simulink model "sim_project_coup"  (R2022a)
settings: Solver=FixedStepAuto  StartTime=0.0  StopTime=5  FixedStep=0.005  RelTol=1e-3
InitFcn:
  | max_thrust = 940/1000 * 10;
  | max_rpm = 13610;
  | k = max_thrust / (max_rpm^2);
  | km = -3.9128e-08;
  | l = 0.3;
  | Izz = 0.026;
values from neighbouring files (symbols this model uses):
  Ixx = Is_sim    [momentofinertia.m]    (also in run_sim_N.m = Is_sim*1.2; run_sim_uns.m = ureal('Ixx',Is_sim,'Percentage',30))
  Iyy = Is_sim    [momentofinertia.m]    (also in run_sim_N.m = Is_sim*0.98; run_sim_uns.m = ureal('Iyy',Is_sim,'Percentage',30))
  K_gain = K_dat(N_sim)    [momentofinertia.m]    (also in run_sim.m = K_dat(N); run_sim_N.m = K_dat(N))
  N = N_sim    (= 2)    [momentofinertia.m]    (also in run_sim.m = 1; run_sim_N.m = i)
  uvars = ufind(mdl)    [run_sim.m]    (also in run_sim_uns.m)
undefined symbols (not defined in the file or in its folder): usample
libraries: slpidlib x5, RCTblocks x5, simulink_extras x3
settings Model: Creator=Kerim  LastModifiedBy=Kerim
settings SolverCC: AlgebraicLoopSolver=TrustRegion
settings DebuggingCC: UnconnectedInputMsg=warning  UnconnectedOutputMsg=warning  UnconnectedLineMsg=warning  SFMachineParentedDataDiag=warning
settings RTWCC: DLArmComputeVersion=19.05

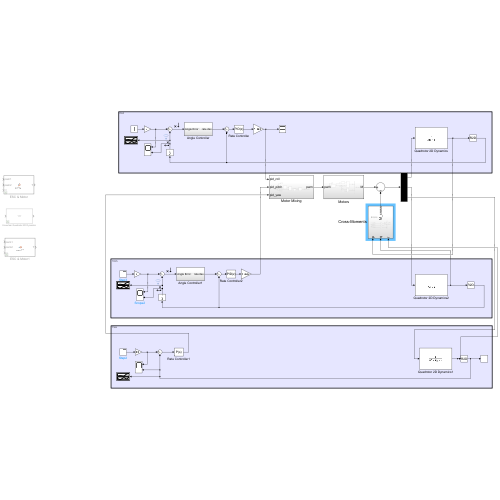
[thumbnail: Simulink's stored preview of the top-level diagram]
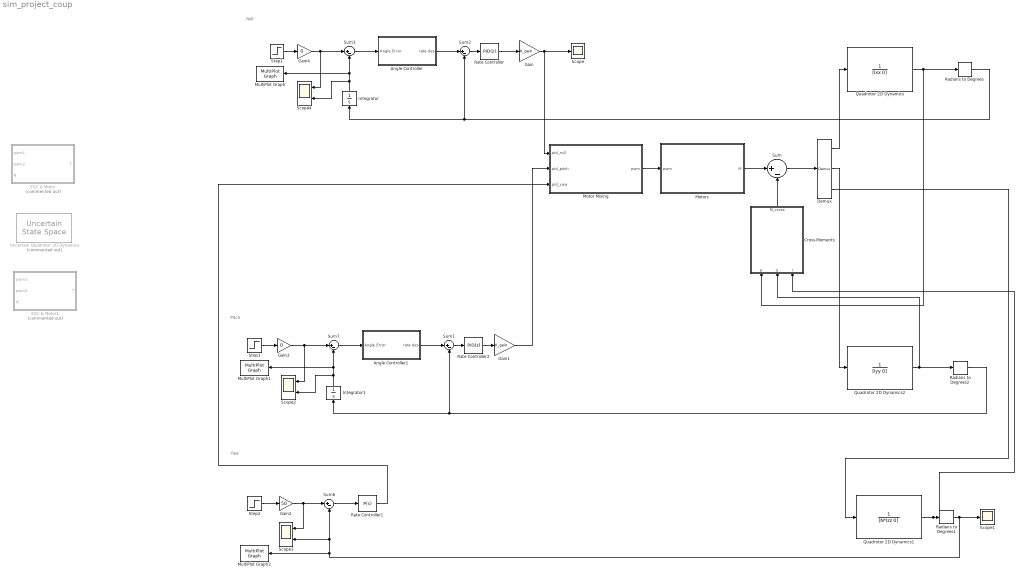
== system sim_project_coup ==
  note: Roll
  note: Yaw
  note: Pitch
  Angle Controller : Subsystem
  Angle Controller1 : Subsystem
  Cross-Moments : Subsystem
  Demux : Demux  Outputs=3
  ESC & Motor : MATLAB Function  Commented=on  TreatAsAtomicUnit=on
  ESC & Motor1 : MATLAB Function  Commented=on  TreatAsAtomicUnit=on
  Gain : Gain  Gain=K_gain
  Gain1 : Gain  Gain=K_gain
  Gain2 : Gain  Gain=50
  Gain3 : Gain  Gain=0
  Gain4 : Gain  Gain=0
  Integrator : Integrator
  Integrator1 : Integrator
  Motor Mixing : Subsystem
  Motors : Subsystem
  MultiPlot Graph : RCTblocks/MultiPlot Graph  Tag=MultiPlot  tmin=0  tmax=5  ymin=-1  ymax=40  Tsamp=-1  vnamesave=multisimout
      settings: SourceProductBaseCode=RC
  MultiPlot Graph1 : RCTblocks/MultiPlot Graph  Tag=MultiPlot  tmin=0  tmax=10  ymin=-1  ymax=2  Tsamp=-1  vnamesave=multisimout1
      settings: SourceProductBaseCode=RC
  MultiPlot Graph2 : RCTblocks/MultiPlot Graph  Tag=MultiPlot  tmin=0  tmax=10  ymin=-1  ymax=2  Tsamp=-1  vnamesave=multisimout2
      settings: SourceProductBaseCode=RC
  Quadrotor 2D Dynamics : TransferFcn  Denominator=[Ixx 0]
  Quadrotor 2D Dynamics1 : TransferFcn  Denominator=[N*Izz 0]
  Quadrotor 2D Dynamics2 : TransferFcn  Denominator=[Iyy 0]
  Radians to Degrees : simulink_extras/Transformations/Radians to Degrees
  Radians to Degrees1 : simulink_extras/Transformations/Radians to Degrees
  Radians to Degrees2 : simulink_extras/Transformations/Radians to Degrees
  Rate Controller : slpidlib/PID Controller  Controller=PID  Form=Parallel  TimeDomain=Discrete-time  UseExternalTs=off  SampleTime=-1  IntegratorMethod=Forward Euler  FilterMethod=Forward Euler  ControllerParametersSource=internal  P=0.48  I=0.08  UseKiTs=off  D=0.008  N=100  UseFilter=on  TunerSelectOption=Transfer Function Based (PID Tuner App)  InitialConditionSource=internal  InitialConditionForIntegrator=0  InitialConditionForFilter=0  DifferentiatorICPrevScaledInput=0  ExternalReset=none  TrackingMode=off  Kt=1  LimitOutput=off  SatLimitsSource=internal  UpperSaturationLimit=inf  LowerSaturationLimit=-inf  LinearizeAsGain=on  AntiWindupMode=none  Kb=1  POutMin=[]  POutMax=[]  IOutMin=[]  IOutMax=[]  DOutMin=[]  DOutMax=[]  NOutMin=[]  NOutMax=[]  SumOutMin=[]  SumOutMax=[]  SaturationOutMin=[]  SaturationOutMax=[]  PParamMin=[]  PParamMax=[]  IParamMin=[]  IParamMax=[]  DParamMin=[]  DParamMax=[]  NParamMin=[]  NParamMax=[]  KbParamMin=[]  KbParamMax=[]  KtParamMin=[]  KtParamMax=[]  KbOutMin=[]  KbOutMax=[]  KtOutMin=[]  KtOutMax=[]  IntegratorOutMin=[]  IntegratorOutMax=[]  FilterOutMin=[]  FilterOutMax=[]  SumI1OutMin=[]  SumI1OutMax=[]  SumI2OutMin=[]  SumI2OutMax=[]  SumI3OutMin=[]  SumI3OutMax=[]  SumI4OutMin=[]  SumI4OutMax=[]  SumDOutMin=[]  SumDOutMax=[]  DifferentiatorOutMin=[]  DifferentiatorOutMax=[]  FilterDiffOutCoefMin=[]  FilterDiffOutCoefMax=[]  ReciprocalOutMin=[]  ReciprocalOutMax=[]  SumDenOutMin=[]  SumDenOutMax=[]  SumNumOutMin=[]  SumNumOutMax=[]  DivideOutMin=[]  DivideOutMax=[]  UdiffTsProdOutMin=[]  UdiffTsProdOutMax=[]  NTsProdOutMin=[]  NTsProdOutMax=[]  UintegralTsProdOutMin=[]  UintegralTsProdOutMax=[]  UngainTsProdOutMin=[]  UngainTsProdOutMax=[]  IntegratorContinuousStateAttributes=''  IntegratorStateMustResolveToSignalObject=off  IntegratorRTWStateStorageClass=Auto  FilterContinuousStateAttributes=''  FilterStateMustResolveToSignalObject=off  FilterRTWStateStorageClass=Auto  ParallelPVariant=InternalParameters  IdealPVariant=Disabled  IVariant=InternalParameters  DVariant=InternalParameters  IntegratorVariant=Discrete  SatVariant=Disabled  AWVariant=Passthrough  PCopyVariant=Disabled  TRVariant=Disabled  FdbkBlocksVariant=Forward  IdealPFdbkVariant=Disabled  SatFdbkVariant=Disabled  DerivativeFilterVariant=ForwardEulerFilter  NVariant=InternalParameters  NCopyVariant=Disabled  FilterICVariant=InternalICsFilter  IntegratorICVariant=InternalICs  ExternalResetVariant=Disabled  TRSumVariant=Passthrough  SumFdbkVariant=Disabled  SumVariant=Sum_PID  TsampFilterVariant=InternalTs  TsampNgainVariant=Passthrough  TsampIntegralVariant=Passthrough  ExternalSaturationOutDataTypeStr=Inherit: Same as second input  aMode=0
  Rate Controller1 : slpidlib/PID Controller  Controller=P  Form=Parallel  TimeDomain=Continuous-time  UseExternalTs=off  SampleTime=-1  IntegratorMethod=Forward Euler  FilterMethod=Forward Euler  ControllerParametersSource=internal  P=5  I=1  UseKiTs=off  D=K_gain*0.06  N=345.128531237038  UseFilter=on  TunerSelectOption=Transfer Function Based (PID Tuner App)  InitialConditionSource=internal  InitialConditionForIntegrator=0  InitialConditionForFilter=0  DifferentiatorICPrevScaledInput=0  ExternalReset=none  TrackingMode=off  Kt=1  LimitOutput=off  SatLimitsSource=internal  UpperSaturationLimit=inf  LowerSaturationLimit=-inf  LinearizeAsGain=on  AntiWindupMode=none  Kb=1  POutMin=[]  POutMax=[]  IOutMin=[]  IOutMax=[]  DOutMin=[]  DOutMax=[]  NOutMin=[]  NOutMax=[]  SumOutMin=[]  SumOutMax=[]  SaturationOutMin=[]  SaturationOutMax=[]  PParamMin=[]  PParamMax=[]  IParamMin=[]  IParamMax=[]  DParamMin=[]  DParamMax=[]  NParamMin=[]  NParamMax=[]  KbParamMin=[]  KbParamMax=[]  KtParamMin=[]  KtParamMax=[]  KbOutMin=[]  KbOutMax=[]  KtOutMin=[]  KtOutMax=[]  IntegratorOutMin=[]  IntegratorOutMax=[]  FilterOutMin=[]  FilterOutMax=[]  SumI1OutMin=[]  SumI1OutMax=[]  SumI2OutMin=[]  SumI2OutMax=[]  SumI3OutMin=[]  SumI3OutMax=[]  SumI4OutMin=[]  SumI4OutMax=[]  SumDOutMin=[]  SumDOutMax=[]  DifferentiatorOutMin=[]  DifferentiatorOutMax=[]  FilterDiffOutCoefMin=[]  FilterDiffOutCoefMax=[]  ReciprocalOutMin=[]  ReciprocalOutMax=[]  SumDenOutMin=[]  SumDenOutMax=[]  SumNumOutMin=[]  SumNumOutMax=[]  DivideOutMin=[]  DivideOutMax=[]  UdiffTsProdOutMin=[]  UdiffTsProdOutMax=[]  NTsProdOutMin=[]  NTsProdOutMax=[]  UintegralTsProdOutMin=[]  UintegralTsProdOutMax=[]  UngainTsProdOutMin=[]  UngainTsProdOutMax=[]  IntegratorContinuousStateAttributes=''  IntegratorStateMustResolveToSignalObject=off  IntegratorRTWStateStorageClass=Auto  FilterContinuousStateAttributes=''  FilterStateMustResolveToSignalObject=off  FilterRTWStateStorageClass=Auto  ParallelPVariant=InternalParameters  IdealPVariant=Disabled  IVariant=Disabled  DVariant=Disabled  IntegratorVariant=Disabled  SatVariant=Disabled  AWVariant=Disabled  PCopyVariant=Disabled  TRVariant=Disabled  FdbkBlocksVariant=Forward  IdealPFdbkVariant=Disabled  SatFdbkVariant=Disabled  DerivativeFilterVariant=Disabled  NVariant=Disabled  NCopyVariant=Disabled_SignalSpec  FilterICVariant=Disabled  IntegratorICVariant=Disabled  ExternalResetVariant=Disabled  TRSumVariant=Passthrough  SumFdbkVariant=Disabled  SumVariant=Passthrough_P  TsampFilterVariant=InternalTs  TsampNgainVariant=Passthrough  TsampIntegralVariant=Disabled_SignalSpec  ExternalSaturationOutDataTypeStr=Inherit: Same as second input  aMode=0
  Rate Controller2 : slpidlib/PID Controller  Controller=PID  Form=Parallel  TimeDomain=Discrete-time  UseExternalTs=off  SampleTime=-1  IntegratorMethod=Forward Euler  FilterMethod=Forward Euler  ControllerParametersSource=internal  P=0.48  I=0.08  UseKiTs=off  D=0.008  N=100  UseFilter=on  TunerSelectOption=Transfer Function Based (PID Tuner App)  InitialConditionSource=internal  InitialConditionForIntegrator=0  InitialConditionForFilter=0  DifferentiatorICPrevScaledInput=0  ExternalReset=none  TrackingMode=off  Kt=1  LimitOutput=off  SatLimitsSource=internal  UpperSaturationLimit=inf  LowerSaturationLimit=-inf  LinearizeAsGain=on  AntiWindupMode=none  Kb=1  POutMin=[]  POutMax=[]  IOutMin=[]  IOutMax=[]  DOutMin=[]  DOutMax=[]  NOutMin=[]  NOutMax=[]  SumOutMin=[]  SumOutMax=[]  SaturationOutMin=[]  SaturationOutMax=[]  PParamMin=[]  PParamMax=[]  IParamMin=[]  IParamMax=[]  DParamMin=[]  DParamMax=[]  NParamMin=[]  NParamMax=[]  KbParamMin=[]  KbParamMax=[]  KtParamMin=[]  KtParamMax=[]  KbOutMin=[]  KbOutMax=[]  KtOutMin=[]  KtOutMax=[]  IntegratorOutMin=[]  IntegratorOutMax=[]  FilterOutMin=[]  FilterOutMax=[]  SumI1OutMin=[]  SumI1OutMax=[]  SumI2OutMin=[]  SumI2OutMax=[]  SumI3OutMin=[]  SumI3OutMax=[]  SumI4OutMin=[]  SumI4OutMax=[]  SumDOutMin=[]  SumDOutMax=[]  DifferentiatorOutMin=[]  DifferentiatorOutMax=[]  FilterDiffOutCoefMin=[]  FilterDiffOutCoefMax=[]  ReciprocalOutMin=[]  ReciprocalOutMax=[]  SumDenOutMin=[]  SumDenOutMax=[]  SumNumOutMin=[]  SumNumOutMax=[]  DivideOutMin=[]  DivideOutMax=[]  UdiffTsProdOutMin=[]  UdiffTsProdOutMax=[]  NTsProdOutMin=[]  NTsProdOutMax=[]  UintegralTsProdOutMin=[]  UintegralTsProdOutMax=[]  UngainTsProdOutMin=[]  UngainTsProdOutMax=[]  IntegratorContinuousStateAttributes=''  IntegratorStateMustResolveToSignalObject=off  IntegratorRTWStateStorageClass=Auto  FilterContinuousStateAttributes=''  FilterStateMustResolveToSignalObject=off  FilterRTWStateStorageClass=Auto  ParallelPVariant=InternalParameters  IdealPVariant=Disabled  IVariant=InternalParameters  DVariant=InternalParameters  IntegratorVariant=Discrete  SatVariant=Disabled  AWVariant=Passthrough  PCopyVariant=Disabled  TRVariant=Disabled  FdbkBlocksVariant=Forward  IdealPFdbkVariant=Disabled  SatFdbkVariant=Disabled  DerivativeFilterVariant=ForwardEulerFilter  NVariant=InternalParameters  NCopyVariant=Disabled  FilterICVariant=InternalICsFilter  IntegratorICVariant=InternalICs  ExternalResetVariant=Disabled  TRSumVariant=Passthrough  SumFdbkVariant=Disabled  SumVariant=Sum_PID  TsampFilterVariant=InternalTs  TsampNgainVariant=Passthrough  TsampIntegralVariant=Passthrough  ExternalSaturationOutDataTypeStr=Inherit: Same as second input  aMode=0
  Scope : Scope
  Scope1 : Scope
  Scope2 : Scope  NumInputPorts=2
  Scope3 : Scope  NumInputPorts=2
  Scope4 : Scope  NumInputPorts=2
  Step1 : Step  SampleTime=0
  Step2 : Step  SampleTime=0
  Step3 : Step  SampleTime=0
  Sum{,1..3,6..7} (6 alike) : Sum  Inputs=|+-
  Uncertain Quadrotor 2D Dynamics : RCTblocks/Uncertain State Space  Tag=USS  Commented=on  USystem=usys  UValue=usample(uvars)  X0=[]  uX0=[]
      settings: SourceProductBaseCode=RC
  wires:
  Rate Controller/1 -> Gain/1
  Angle Controller/1(rate des) -> Sum2/1
  Sum2/1 -> Rate Controller/1
  Sum3/1 -> Angle Controller/1(Angle Error)
  Step1/1 -> Gain4/1
  Quadrotor 2D Dynamics1/1 -> Radians to Degrees1/1, Cross-Moments/3(r)
  Sum6/1 -> Rate Controller1/1
  Radians to Degrees1/1 -> Sum6/2, Scope3/2, MultiPlot Graph2/1, Scope1/1
  Step2/1 -> Gain2/1
  Radians to Degrees/1 -> Sum2/2, Integrator/1
  Integrator/1 -> Scope4/2, Sum3/2, MultiPlot Graph/1
  Quadrotor 2D Dynamics/1 -> Radians to Degrees/1, Cross-Moments/1(p)
  Quadrotor 2D Dynamics2/1 -> Radians to Degrees2/1, Cross-Moments/2(q)
  Integrator1/1 -> Scope2/2, Sum7/2, MultiPlot Graph1/1
  Radians to Degrees2/1 -> Sum1/2, Integrator1/1
  Angle Controller1/1(rate des) -> Sum1/1
  Sum7/1 -> Angle Controller1/1(Angle Error)
  Sum1/1 -> Rate Controller2/1
  Step3/1 -> Gain3/1
  Rate Controller2/1 -> Gain1/1
  Gain/1 -> Scope/1, Motor Mixing/1(pid_roll)
  Gain1/1 -> Motor Mixing/2(pid_pitch)
  Rate Controller1/1 -> Motor Mixing/3(pid_yaw)
  Motor Mixing/1(pwm) -> Motors/1(pwm)
  Motors/1(M) -> Sum/1
  Sum/1 -> Demux/1
  Demux/1 -> Quadrotor 2D Dynamics/1
  Demux/2 -> Quadrotor 2D Dynamics2/1
  Demux/3 -> Quadrotor 2D Dynamics1/1
  Gain2/1 -> Scope3/1, Sum6/1
  Gain3/1 -> Scope2/1, Sum7/1
  Gain4/1 -> Scope4/1, Sum3/1
  Cross-Moments/1(M_cross) -> Sum/2

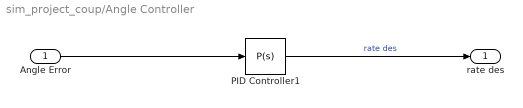
== system sim_project_coup/Angle Controller ==
  Angle Error : Inport
  PID Controller1 : slpidlib/PID Controller  Controller=P  Form=Parallel  TimeDomain=Continuous-time  UseExternalTs=off  SampleTime=-1  IntegratorMethod=Forward Euler  FilterMethod=Forward Euler  ControllerParametersSource=internal  P=4.5  I=0  UseKiTs=off  D=0  N=100  UseFilter=on  TunerSelectOption=Transfer Function Based (PID Tuner App)  InitialConditionSource=internal  InitialConditionForIntegrator=0  InitialConditionForFilter=0  DifferentiatorICPrevScaledInput=0  ExternalReset=none  TrackingMode=off  Kt=1  LimitOutput=off  SatLimitsSource=internal  UpperSaturationLimit=inf  LowerSaturationLimit=-inf  LinearizeAsGain=on  AntiWindupMode=none  Kb=1  POutMin=[]  POutMax=[]  IOutMin=[]  IOutMax=[]  DOutMin=[]  DOutMax=[]  NOutMin=[]  NOutMax=[]  SumOutMin=[]  SumOutMax=[]  SaturationOutMin=[]  SaturationOutMax=[]  PParamMin=[]  PParamMax=[]  IParamMin=[]  IParamMax=[]  DParamMin=[]  DParamMax=[]  NParamMin=[]  NParamMax=[]  KbParamMin=[]  KbParamMax=[]  KtParamMin=[]  KtParamMax=[]  KbOutMin=[]  KbOutMax=[]  KtOutMin=[]  KtOutMax=[]  IntegratorOutMin=[]  IntegratorOutMax=[]  FilterOutMin=[]  FilterOutMax=[]  SumI1OutMin=[]  SumI1OutMax=[]  SumI2OutMin=[]  SumI2OutMax=[]  SumI3OutMin=[]  SumI3OutMax=[]  SumI4OutMin=[]  SumI4OutMax=[]  SumDOutMin=[]  SumDOutMax=[]  DifferentiatorOutMin=[]  DifferentiatorOutMax=[]  FilterDiffOutCoefMin=[]  FilterDiffOutCoefMax=[]  ReciprocalOutMin=[]  ReciprocalOutMax=[]  SumDenOutMin=[]  SumDenOutMax=[]  SumNumOutMin=[]  SumNumOutMax=[]  DivideOutMin=[]  DivideOutMax=[]  UdiffTsProdOutMin=[]  UdiffTsProdOutMax=[]  NTsProdOutMin=[]  NTsProdOutMax=[]  UintegralTsProdOutMin=[]  UintegralTsProdOutMax=[]  UngainTsProdOutMin=[]  UngainTsProdOutMax=[]  IntegratorContinuousStateAttributes=''  IntegratorStateMustResolveToSignalObject=off  IntegratorRTWStateStorageClass=Auto  FilterContinuousStateAttributes=''  FilterStateMustResolveToSignalObject=off  FilterRTWStateStorageClass=Auto  ParallelPVariant=InternalParameters  IdealPVariant=Disabled  IVariant=Disabled  DVariant=Disabled  IntegratorVariant=Disabled  SatVariant=Disabled  AWVariant=Disabled  PCopyVariant=Disabled  TRVariant=Disabled  FdbkBlocksVariant=Forward  IdealPFdbkVariant=Disabled  SatFdbkVariant=Disabled  DerivativeFilterVariant=Disabled  NVariant=Disabled  NCopyVariant=Disabled_SignalSpec  FilterICVariant=Disabled  IntegratorICVariant=Disabled  ExternalResetVariant=Disabled  TRSumVariant=Passthrough  SumFdbkVariant=Disabled  SumVariant=Passthrough_P  TsampFilterVariant=InternalTs  TsampNgainVariant=Passthrough  TsampIntegralVariant=Disabled_SignalSpec  ExternalSaturationOutDataTypeStr=Inherit: Same as second input  aMode=0
  rate des : Outport
  wires:
  Angle Error/1 -> PID Controller1/1
  PID Controller1/1 -> rate des/1  "rate des"

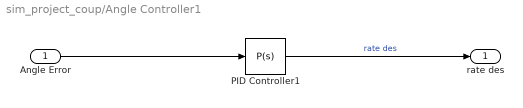
== system sim_project_coup/Angle Controller1 ==
  Angle Error : Inport
  PID Controller1 : slpidlib/PID Controller  Controller=P  Form=Parallel  TimeDomain=Continuous-time  UseExternalTs=off  SampleTime=-1  IntegratorMethod=Forward Euler  FilterMethod=Forward Euler  ControllerParametersSource=internal  P=4.5  I=0  UseKiTs=off  D=0  N=100  UseFilter=on  TunerSelectOption=Transfer Function Based (PID Tuner App)  InitialConditionSource=internal  InitialConditionForIntegrator=0  InitialConditionForFilter=0  DifferentiatorICPrevScaledInput=0  ExternalReset=none  TrackingMode=off  Kt=1  LimitOutput=off  SatLimitsSource=internal  UpperSaturationLimit=inf  LowerSaturationLimit=-inf  LinearizeAsGain=on  AntiWindupMode=none  Kb=1  POutMin=[]  POutMax=[]  IOutMin=[]  IOutMax=[]  DOutMin=[]  DOutMax=[]  NOutMin=[]  NOutMax=[]  SumOutMin=[]  SumOutMax=[]  SaturationOutMin=[]  SaturationOutMax=[]  PParamMin=[]  PParamMax=[]  IParamMin=[]  IParamMax=[]  DParamMin=[]  DParamMax=[]  NParamMin=[]  NParamMax=[]  KbParamMin=[]  KbParamMax=[]  KtParamMin=[]  KtParamMax=[]  KbOutMin=[]  KbOutMax=[]  KtOutMin=[]  KtOutMax=[]  IntegratorOutMin=[]  IntegratorOutMax=[]  FilterOutMin=[]  FilterOutMax=[]  SumI1OutMin=[]  SumI1OutMax=[]  SumI2OutMin=[]  SumI2OutMax=[]  SumI3OutMin=[]  SumI3OutMax=[]  SumI4OutMin=[]  SumI4OutMax=[]  SumDOutMin=[]  SumDOutMax=[]  DifferentiatorOutMin=[]  DifferentiatorOutMax=[]  FilterDiffOutCoefMin=[]  FilterDiffOutCoefMax=[]  ReciprocalOutMin=[]  ReciprocalOutMax=[]  SumDenOutMin=[]  SumDenOutMax=[]  SumNumOutMin=[]  SumNumOutMax=[]  DivideOutMin=[]  DivideOutMax=[]  UdiffTsProdOutMin=[]  UdiffTsProdOutMax=[]  NTsProdOutMin=[]  NTsProdOutMax=[]  UintegralTsProdOutMin=[]  UintegralTsProdOutMax=[]  UngainTsProdOutMin=[]  UngainTsProdOutMax=[]  IntegratorContinuousStateAttributes=''  IntegratorStateMustResolveToSignalObject=off  IntegratorRTWStateStorageClass=Auto  FilterContinuousStateAttributes=''  FilterStateMustResolveToSignalObject=off  FilterRTWStateStorageClass=Auto  ParallelPVariant=InternalParameters  IdealPVariant=Disabled  IVariant=Disabled  DVariant=Disabled  IntegratorVariant=Disabled  SatVariant=Disabled  AWVariant=Disabled  PCopyVariant=Disabled  TRVariant=Disabled  FdbkBlocksVariant=Forward  IdealPFdbkVariant=Disabled  SatFdbkVariant=Disabled  DerivativeFilterVariant=Disabled  NVariant=Disabled  NCopyVariant=Disabled_SignalSpec  FilterICVariant=Disabled  IntegratorICVariant=Disabled  ExternalResetVariant=Disabled  TRSumVariant=Passthrough  SumFdbkVariant=Disabled  SumVariant=Passthrough_P  TsampFilterVariant=InternalTs  TsampNgainVariant=Passthrough  TsampIntegralVariant=Disabled_SignalSpec  ExternalSaturationOutDataTypeStr=Inherit: Same as second input  aMode=0
  rate des : Outport
  wires:
  Angle Error/1 -> PID Controller1/1
  PID Controller1/1 -> rate des/1  "rate des"

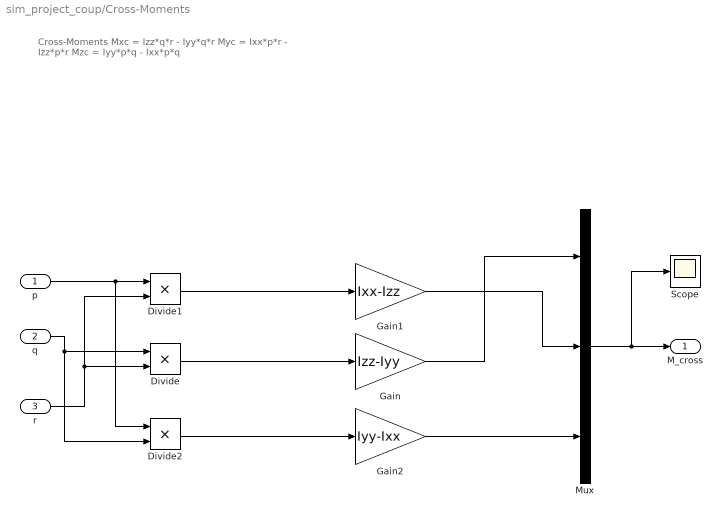
== system sim_project_coup/Cross-Moments ==
  note: Cross-Moments
      | Mxc = Izz*q*r - Iyy*q*r
      | Myc = Ixx*p*r - Izz*p*r
      | Mzc = Iyy*p*q - Ixx*p*q
  p : Inport
  q : Inport  Port=2
  r : Inport  Port=3
  Divide : Product  Inputs=**
  Divide1 : Product  Inputs=**
  Divide2 : Product  Inputs=**
  Gain : Gain  Gain=Izz-Iyy
  Gain1 : Gain  Gain=Ixx-Izz
  Gain2 : Gain  Gain=Iyy-Ixx
  Mux : Mux  Inputs=3
  Scope : Scope
  M_cross : Outport
  wires:
  q/1 -> Divide2/2, Divide/1
  r/1 -> Divide1/2, Divide/2
  Divide/1 -> Gain/1
  p/1 -> Divide2/1, Divide1/1
  Divide1/1 -> Gain1/1
  Divide2/1 -> Gain2/1
  Gain/1 -> Mux/1
  Gain1/1 -> Mux/2
  Gain2/1 -> Mux/3
  Mux/1 -> Scope/1, M_cross/1

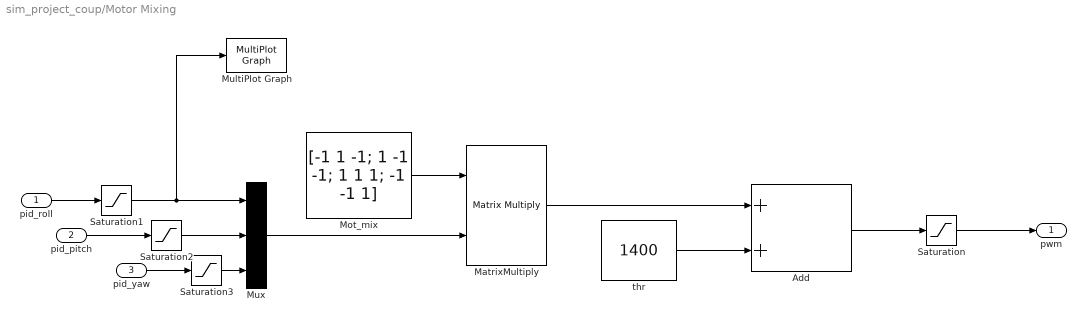
== system sim_project_coup/Motor Mixing ==
  pid_roll : Inport
  pid_pitch : Inport  Port=2
  pid_yaw : Inport  Port=3
  Add : Sum
  MatrixMultiply : Product  Multiplication=Matrix(*)
  Mot_mix : Constant  Value=[-1 1 -1; 1 -1 -1; 1 1 1; -1 -1 1]
  MultiPlot Graph : RCTblocks/MultiPlot Graph  Tag=MultiPlot  tmin=0  tmax=5  ymin=-400  ymax=400  Tsamp=-1  vnamesave=multisimout
      settings: SourceProductBaseCode=RC
  Mux : Mux  Inputs=3
  Saturation : Saturate  UpperLimit=2000  LowerLimit=1100
  Saturation1 : Saturate  UpperLimit=300  LowerLimit=-300
  Saturation2 : Saturate  UpperLimit=300  LowerLimit=-300
  Saturation3 : Saturate  UpperLimit=300  LowerLimit=-300
  thr : Constant  Value=1400
  pwm : Outport
  wires:
  thr/1 -> Add/2
  pid_pitch/1 -> Saturation2/1
  MatrixMultiply/1 -> Add/1
  Mot_mix/1 -> MatrixMultiply/1
  pid_roll/1 -> Saturation1/1
  Mux/1 -> MatrixMultiply/2
  Add/1 -> Saturation/1
  pid_yaw/1 -> Saturation3/1
  Saturation/1 -> pwm/1
  Saturation1/1 -> MultiPlot Graph/1, Mux/1
  Saturation2/1 -> Mux/2
  Saturation3/1 -> Mux/3

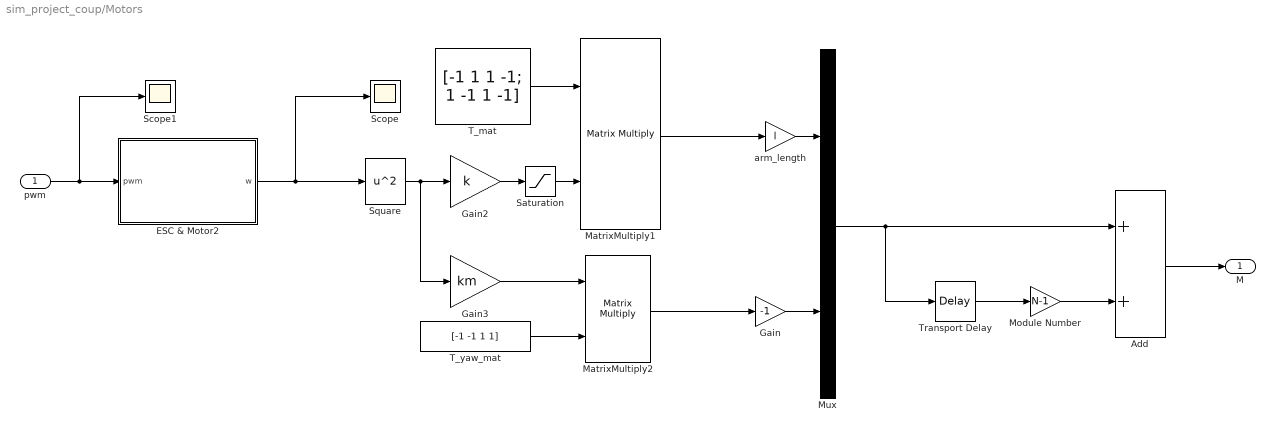
== system sim_project_coup/Motors ==
  pwm : Inport
  Add : Sum
  ESC & Motor2 : MATLAB Function  TreatAsAtomicUnit=on
  Gain : Gain  Gain=-1
  Gain2 : Gain  Gain=k
  Gain3 : Gain  Gain=km
  MatrixMultiply1 : Product  Multiplication=Matrix(*)
  MatrixMultiply2 : Product  Multiplication=Matrix(*)
  Module Number : Gain  Gain=N-1
  Mux : Mux  Inputs=2
  Saturation : Saturate  UpperLimit=10  LowerLimit=0
  Scope : Scope
  Scope1 : Scope
  Square : Math  Operator=square
  T_mat : Constant  Value=[-1 1 1 -1; 1 -1 1 -1]
  T_yaw_mat : Constant  Value=[-1 -1 1 1]
  Transport Delay : TransportDelay  PadeOrder=2
  arm_length : Gain  Gain=l
  M : Outport
  wires:
  MatrixMultiply1/1 -> arm_length/1
  ESC & Motor2/1(w) -> Scope/1, Square/1
  Gain2/1 -> Saturation/1
  T_mat/1 -> MatrixMultiply1/1
  T_yaw_mat/1 -> MatrixMultiply2/2
  Square/1 -> Gain2/1, Gain3/1
  Gain3/1 -> MatrixMultiply2/1
  pwm/1 -> Scope1/1, ESC & Motor2/1(pwm)
  MatrixMultiply2/1 -> Gain/1
  arm_length/1 -> Mux/1
  Saturation/1 -> MatrixMultiply1/2
  Gain/1 -> Mux/2
  Mux/1 -> Transport Delay/1, Add/1
  Transport Delay/1 -> Module Number/1
  Module Number/1 -> Add/2
  Add/1 -> M/1

== matlab function sim_project_coup/ESC & Motor1 ==
  data: pwm1 input; T output; pwm2 input; N input
function T = pwm2T(pwm1,pwm2,N)
max_thrust = 940/1000 * 10;
max_rpm = 13610;
k = max_thrust / (max_rpm^2)*0.05;
l = 0.15;
w1 = (pwm1 - 1000) * (max_rpm - 0) / (2000 - 1000) + 0;
w2 = (pwm2 - 1000) * (max_rpm - 0) / (2000 - 1000) + 0;


M1 = k*w1^2; M2=k*w2^2;

T = N*2*(M2-M1);

== matlab function sim_project_coup/ESC & Motor ==
  data: pwm1 input; T output; pwm2 input; N input
function T = pwm2T(pwm1,pwm2,N)
max_thrust = 940/1000 * 10;
max_rpm = 13610;
k = max_thrust / (max_rpm^2);
l = 0.2;
w1 = (pwm1 - 1000) * (max_rpm - 0) / (2000 - 1000) + 0;
w2 = (pwm2 - 1000) * (max_rpm - 0) / (2000 - 1000) + 0;


F1 = k*w1^2; F2=k*w2^2;

T = N*2*(F2-F1)*l;

== matlab function sim_project_coup/Motors/ESC & Motor2 ==
  data: pwm input; w output
function w = pwm2w(pwm)
max_thrust = 940/1000 * 10;
max_rpm = 13610;
k = max_thrust / (max_rpm^2);
l = 0.3;
w1 = (pwm(1) - 1000) * (max_rpm - 0) / (2000 - 1000) + 0;
w2 = (pwm(2) - 1000) * (max_rpm - 0) / (2000 - 1000) + 0;
w3 = (pwm(3) - 1000) * (max_rpm - 0) / (2000 - 1000) + 0;
w4 = (pwm(4) - 1000) * (max_rpm - 0) / (2000 - 1000) + 0;

w = [w1 w2 w3 w4]';

%F1 = k*w1^2; F2=k*w2^2;
%T = N*2*(F2-F1)*l;
